simulink model "Reverberator"  (R2018a)
settings: Solver=VariableStepAuto  StartTime=0.0  StopTime=30.0  RelTol=1e-3
libraries: dspsrcs4 x1
settings Model: Creator=Manuel  LastModifiedBy=Manuel

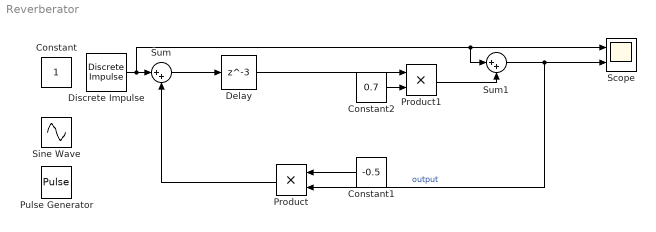
== system Reverberator ==
  Constant : Constant
  Constant1 : Constant  Value=-0.5
  Constant2 : Constant  Value=0.7
  Delay : Delay  DelayLength=3  InitialCondition=0
  Discrete Impulse : dspsrcs4/Discrete  Impulse  Delay=0  SampleTime=1  FrameSample=1  OutputFrames=off  dataType=double  isSigned=on  wordLen=16  udDataType=sfix(16)  fracBitsMode=Best precision  numFracBits=15  OutDataTypeStr=double  LastOutDataTypeStr=double
  Product : Product
  Product1 : Product
  Pulse Generator : DiscretePulseGenerator  PulseType=Time based  Period=10  PulseWidth=5
  Scope : Scope  NumInputPorts=2
  Sine Wave : Sin  SampleTime=0
  Sum : Sum  Inputs=|++
  Sum1 : Sum  Inputs=|++
  wires:
  Delay/1 -> Product1/1
  Sum/1 -> Delay/1
  Product/1 -> Sum/2
  Constant1/1 -> Product/1
  Constant2/1 -> Product1/2
  Product1/1 -> Sum1/2
  Sum1/1 -> Scope/2, Product/2  "output"
  Discrete Impulse/1 -> Sum1/1, Scope/1, Sum/1
